simulink model "Yaw2doF"  (R2019b)
settings: Solver=VariableStepAuto  StartTime=0.0  StopTime=10.0  RelTol=1e-3
undefined symbols (not defined in the file): Dt, F_limit, Jy, k_py, k_yaw
settings Model: Creator=lbend  LastModifiedBy=lbend

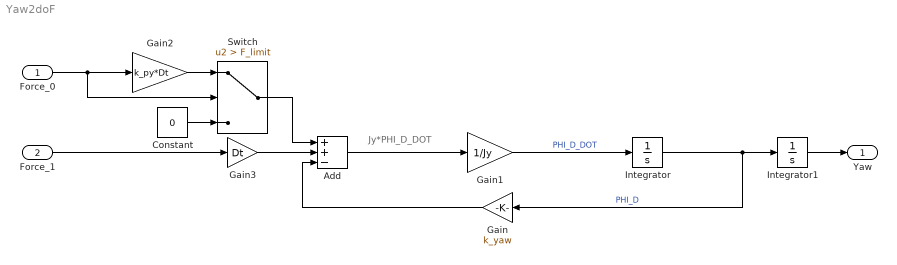
== system Yaw2doF ==
  note: Jy*PHI_D_DOT
  Force_0 : Inport
  "Force_1 " : Inport  Port=2
  Add : Sum  Inputs=++-
  Constant : Constant  Value=0
  Gain : Gain  Gain=k_yaw
  Gain1 : Gain  Gain=1/Jy
  Gain2 : Gain  Gain=k_py*Dt
  Gain3 : Gain  Gain=Dt
  Integrator : Integrator
  Integrator1 : Integrator
  Switch : Switch  Criteria=u2 > Threshold  Threshold=F_limit
  Yaw : Outport
  wires:
  Gain2/1 -> Switch/1
  Switch/1 -> Add/1
  Gain3/1 -> Add/2
  Gain1/1 -> Integrator/1  "PHI_D_DOT"
  Force_0/1 -> Switch/2, Gain2/1
  Add/1 -> Gain1/1
  Gain/1 -> Add/3
  Integrator/1 -> Gain/1, Integrator1/1  "PHI_D"
  Integrator1/1 -> Yaw/1
  "Force_1 "/1 -> Gain3/1
  Constant/1 -> Switch/3
